simulink model "mMaskedSubsystem_g790093"  (Simulink 8.0)
settings: Solver=FixedStepDiscrete  SolverMode=SingleTasking  StartTime=0  StopTime=10  RelTol=1e-3
settings Model: Creator=demxk5w5  LastModifiedBy=hungdang
settings DataIOCC: SignalLoggingSaveFormat=ModelDataLogs  SaveOutput=off  SignalLogging=off  SaveTime=off
settings OptimizationCC: BlockReduction=off  ConditionallyExecuteInputs=off  InlineParams=on  InitFltsAndDblsToZero=on  EfficientMapNaN2IntZero=off
settings DebuggingCC: AlgebraicLoopMsg=error  SingleTaskRateTransMsg=error  FcnCallInpInsideContextMsg=Use local settings
settings HardwareCC: ProdHWDeviceType=ASIC/FPGA->ASIC/FPGA  ProdEqTarget=off
settings SFSimCC: SFSimEnableDebug=off  SimParseCustomCode=off
settings GRTTargetCC: CombineOutputUpdateFcns=off  GRTInterface=on

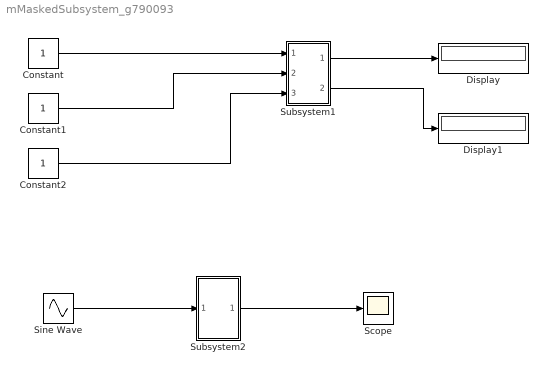
== system mMaskedSubsystem_g790093 ==
  Constant : Constant  OutDataTypeStr=fixdt(0,12,0)  SampleTime=1
  Constant1 : Constant  OutDataTypeStr=boolean  SampleTime=1
  Constant2 : Constant  OutDataTypeStr=boolean  SampleTime=1
  Display : Display
  Display1 : Display
  Scope : Scope
  Sine Wave : Sin  SampleTime=0
  Subsystem1 : Subsystem
  Subsystem2 : Subsystem  TreatAsAtomicUnit=on  mask{k=1}
      mask prompts: k "Unused variable"
  wires:
  Constant/1 -> Subsystem1/1(In1)
  Constant1/1 -> Subsystem1/2(In2)
  Constant2/1 -> Subsystem1/3(In3)
  Subsystem1/1(Out1) -> Display/1
  Subsystem1/2(Out2) -> Display1/1
  Sine Wave/1 -> Subsystem2/1(In1)
  Subsystem2/1(Out1) -> Scope/1

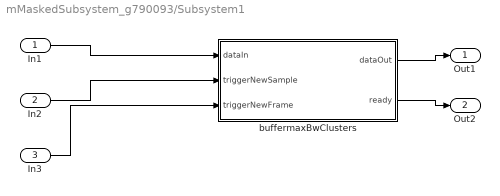
== system mMaskedSubsystem_g790093/Subsystem1 ==
  In1 : Inport
  In2 : Inport  Port=2
  In3 : Inport  Port=3
  buffermaxBwClusters : Subsystem  TreatAsAtomicUnit=on
      mask Description: Test
  Out1 : Outport
  Out2 : Outport  Port=2
  wires:
  In1/1 -> buffermaxBwClusters/1(dataIn)
  In3/1 -> buffermaxBwClusters/3(triggerNewFrame)
  buffermaxBwClusters/1(dataOut) -> Out1/1
  buffermaxBwClusters/2(ready) -> Out2/1
  In2/1 -> buffermaxBwClusters/2(triggerNewSample)

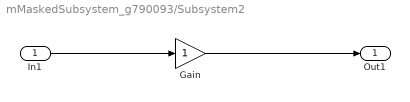
== system mMaskedSubsystem_g790093/Subsystem2 ==
  In1 : Inport
  Gain : Gain
  Out1 : Outport
  wires:
  In1/1 -> Gain/1
  Gain/1 -> Out1/1

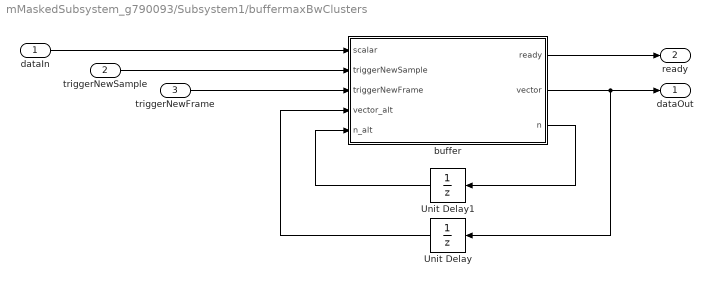
== system mMaskedSubsystem_g790093/Subsystem1/buffermaxBwClusters ==
  dataIn : Inport
  triggerNewSample : Inport  Port=2
  triggerNewFrame : Inport  Port=3
  Unit Delay : UnitDelay  X0=1  SampleTime=-1
  Unit Delay1 : UnitDelay  X0=1  SampleTime=-1
  buffer : MATLAB Function  TreatAsAtomicUnit=on
  dataOut : Outport
  ready : Outport  Port=2
  wires:
  triggerNewFrame/1 -> buffer/3(triggerNewFrame)
  triggerNewSample/1 -> buffer/2(triggerNewSample)
  buffer/2(vector) -> dataOut/1, Unit Delay/1
  buffer/1(ready) -> ready/1
  dataIn/1 -> buffer/1(scalar)
  buffer/3(n) -> Unit Delay1/1
  Unit Delay1/1 -> buffer/5(n_alt)
  Unit Delay/1 -> buffer/4(vector_alt)

== matlab function Subsystem1/buffermaxBwClusters/buffer ==
  settings: fimath=|
      | fimath(...
      | 'RoundMode', 'nearest',...
      | 'OverflowMode', 'wrap',...
      | 'ProductMode', 'KeepLSB', 'ProductWordLength', 32,...
      | 'SumMode', 'KeepLSB', 'SumWordLength', 32,...
      | 'CastBeforeSum', true)
  data: scalar input boolean; triggerNewSample input boolean; triggerNewFrame input boolean; vector_alt input fixdt(0,12,0); n_alt input uint8; ready output boolean; vector output double; n output uint8
function [ready,vector,n] = fcn(scalar,triggerNewSample,triggerNewFrame,vector_alt,n_alt)
% This block supports the Embedded MATLAB subset.
% See the help menu for details. 
% calc index / ready-flag, add new scalar to vector
if triggerNewFrame == 1
    n = uint8(1);
    ready = false;
    vector = fi(zeros(64,1),numerictype(scalar),fimath(scalar));
elseif n_alt <= 64
    vector = vector_alt;
    n = n_alt;
    if triggerNewSample
        vector (n,1) = scalar;
        n = n_alt + 1;
    end
    ready = false;
else
    vector = vector_alt;
    n = n_alt;
    ready = true;
end
